simulink model "control_mkb"  (R2018a)
settings: Solver=VariableStepAuto  StartTime=0.0  StopTime=100  RelTol=1e-3
InitFcn:
  | m=10; M=m*0.7;
  | b=4; B=b*0.85;
  | k=5; K=k*1.20;
  | Kp=-4.6*1;
  | Kv=0.5*Kp*0;
settings Model: Creator=Owner  LastModifiedBy=Owner

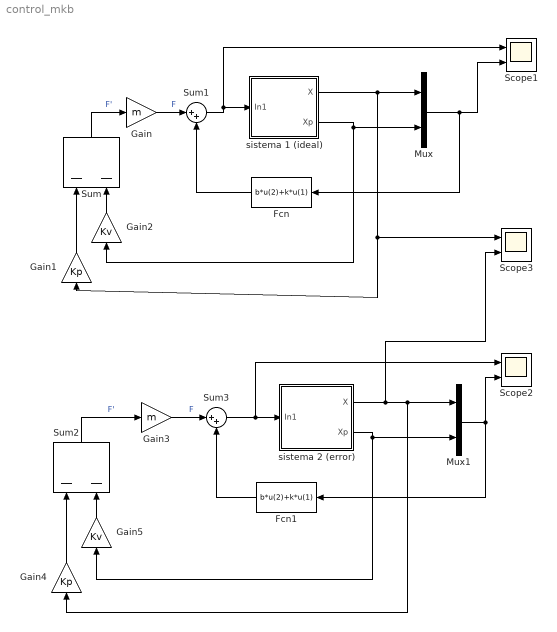
== system control_mkb ==
  Fcn : Fcn  Expr=b*u(2)+k*u(1)
  Fcn1 : Fcn  Expr=b*u(2)+k*u(1)
  Gain : Gain  Gain=m
  Gain1 : Gain  Gain=Kp
  Gain2 : Gain  Gain=Kv
  Gain3 : Gain  Gain=m
  Gain4 : Gain  Gain=Kp
  Gain5 : Gain  Gain=Kv
  Mux : Mux  Inputs=2
  Mux1 : Mux  Inputs=2
  Scope1 : Scope  NumInputPorts=2
  Scope2 : Scope  NumInputPorts=2
  Scope3 : Scope  NumInputPorts=2
  Sum : Sum  Inputs=--
  Sum1 : Sum  Inputs=|++
  Sum2 : Sum  Inputs=--
  Sum3 : Sum  Inputs=|++
  sistema 1 (ideal) : Subsystem
  sistema 2 (error) : Subsystem
  wires:
  Gain1/1 -> Sum/1
  Gain2/1 -> Sum/2
  Sum/1 -> Gain/1  "F'"
  Gain/1 -> Sum1/1  "F"
  sistema 1 (ideal)/2(Xp) -> Gain2/1, Mux/2
  Mux/1 -> Scope1/2, Fcn/1
  sistema 1 (ideal)/1(X) -> Gain1/1, Scope3/1, Mux/1
  Sum1/1 -> Scope1/1, sistema 1 (ideal)/1(In1)
  Fcn/1 -> Sum1/2
  Gain4/1 -> Sum2/1
  Gain3/1 -> Sum3/1  "F"
  Sum3/1 -> Scope2/1, sistema 2 (error)/1(In1)
  Sum2/1 -> Gain3/1  "F'"
  Fcn1/1 -> Sum3/2
  sistema 2 (error)/2(Xp) -> Gain5/1, Mux1/2
  Mux1/1 -> Scope2/2, Fcn1/1
  sistema 2 (error)/1(X) -> Scope3/2, Mux1/1, Gain4/1
  Gain5/1 -> Sum2/2

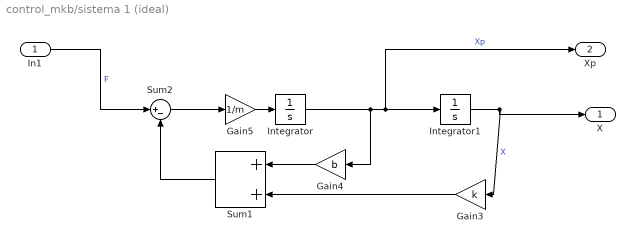
== system control_mkb/sistema 1 (ideal) ==
  In1 : Inport
  Gain3 : Gain  Gain=k
  Gain4 : Gain  Gain=b
  Gain5 : Gain  Gain=1/m
  Integrator : Integrator  InitialCondition=10
  Integrator1 : Integrator
  Sum1 : Sum
  Sum2 : Sum  Inputs=|+-
  X : Outport
  Xp : Outport  Port=2
  wires:
  Integrator/1 -> Gain4/1, Xp/1, Integrator1/1  "Xp"
  Gain4/1 -> Sum1/1
  Integrator1/1 -> X/1, Gain3/1  "X"
  In1/1 -> Sum2/1  "F"
  Sum2/1 -> Gain5/1
  Gain5/1 -> Integrator/1
  Gain3/1 -> Sum1/2
  Sum1/1 -> Sum2/2

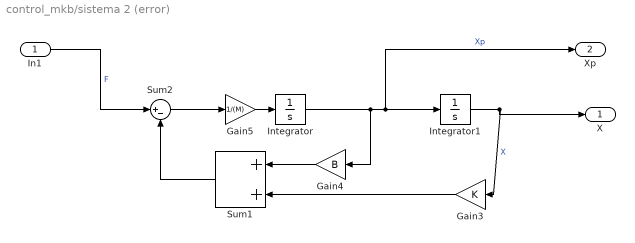
== system control_mkb/sistema 2 (error) ==
  In1 : Inport
  Gain3 : Gain  Gain=K
  Gain4 : Gain  Gain=B
  Gain5 : Gain  Gain=1/(M)
  Integrator : Integrator  InitialCondition=10
  Integrator1 : Integrator
  Sum1 : Sum
  Sum2 : Sum  Inputs=|+-
  X : Outport
  Xp : Outport  Port=2
  wires:
  Integrator/1 -> Gain4/1, Xp/1, Integrator1/1  "Xp"
  Gain4/1 -> Sum1/1
  Integrator1/1 -> X/1, Gain3/1  "X"
  In1/1 -> Sum2/1  "F"
  Sum2/1 -> Gain5/1
  Gain5/1 -> Integrator/1
  Gain3/1 -> Sum1/2
  Sum1/1 -> Sum2/2
